simulink model "quad_control"  (R2014b)
settings: Solver=ode3  StartTime=0.0  StopTime=100  FixedStep=0.01  RelTol=1e-3
values from neighbouring files (symbols this model uses):
  g = 9.8    [init.m]
  m = 0.18    [init.m]
undefined symbols (not defined in the file or in its folder): attitude_control, commanded_cord, model, position_control
libraries: simulink x2
settings Model: CovSFcnEnable=on  Creator=smishra  LastModifiedBy=smishra
settings DebuggingCC: SolverPrmCheckMsg=none  FrameProcessingCompatibilityMsg=error

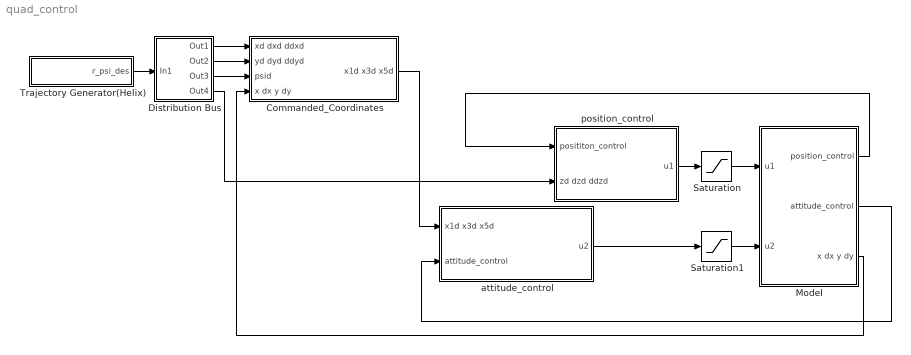
== system quad_control ==
  Commanded_Coordinates : Subsystem
  Distribution Bus : Subsystem
  Model : Subsystem
  Saturation : Saturate  UpperLimit=2*m*g  LowerLimit=0
  Saturation1 : Saturate  UpperLimit=0.2  LowerLimit=-0.2
  Trajectory Generator(Helix) : Subsystem
  attitude_control : Subsystem
  position_control : Subsystem
  wires:
  Model/1(position_control) -> position_control/1(posititon_control)
  Commanded_Coordinates/1(x1d x3d x5d) -> attitude_control/1(x1d x3d x5d)
  Model/2(attitude_control) -> attitude_control/2(attitude_control)
  Model/3(x dx y dy) -> Commanded_Coordinates/4(x dx y dy)
  position_control/1(u1) -> Saturation/1
  Saturation/1 -> Model/1(u1)
  Saturation1/1 -> Model/2(u2)
  attitude_control/1(u2) -> Saturation1/1
  Trajectory Generator(Helix)/1(r_psi_des) -> Distribution Bus/1(In1)
  Distribution Bus/1(Out1) -> Commanded_Coordinates/1(xd dxd ddxd)
  Distribution Bus/2(Out2) -> Commanded_Coordinates/2(yd dyd ddyd)
  Distribution Bus/3(Out3) -> Commanded_Coordinates/3(psid)
  Distribution Bus/4(Out4) -> position_control/2(zd dzd ddzd)

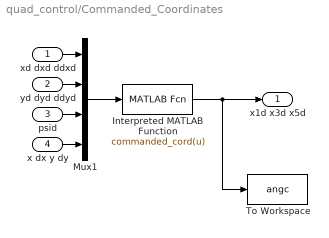
== system quad_control/Commanded_Coordinates ==
  xd dxd ddxd : Inport
  yd dyd ddyd : Inport  Port=2
  psid : Inport  Port=3
  x dx y dy : Inport  Port=4
  Interpreted MATLAB Function : MATLABFcn  MATLABFcn=commanded_cord(u)  OutputDimensions=3
  Mux1 : Mux
  To Workspace : ToWorkspace  VariableName=angc  SampleTime=-1
  x1d x3d x5d : Outport
  wires:
  yd dyd ddyd/1 -> Mux1/2
  xd dxd ddxd/1 -> Mux1/1
  psid/1 -> Mux1/3
  Interpreted MATLAB Function/1 -> To Workspace/1, x1d x3d x5d/1
  Mux1/1 -> Interpreted MATLAB Function/1
  x dx y dy/1 -> Mux1/4

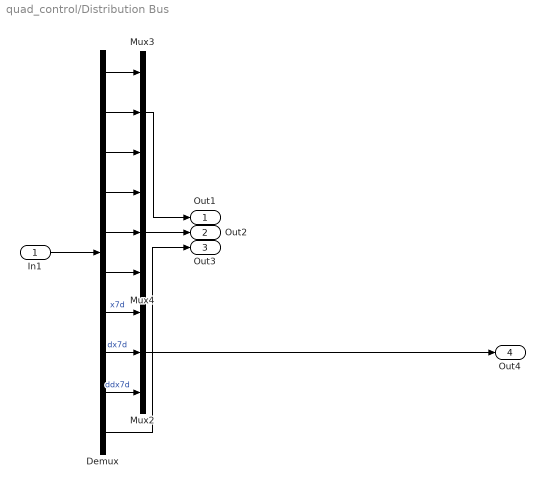
== system quad_control/Distribution Bus ==
  In1 : Inport
  Demux : Demux  Outputs=10
  Mux2 : Mux  Inputs=3
  Mux3 : Mux  Inputs=3
  Mux4 : Mux  Inputs=3
  Out1 : Outport
  Out2 : Outport  Port=2
  Out3 : Outport  Port=3
  Out4 : Outport  Port=4
  wires:
  Demux/10 -> Out3/1
  Mux4/1 -> Out2/1
  Mux3/1 -> Out1/1
  In1/1 -> Demux/1
  Demux/5 -> Mux4/2
  Demux/6 -> Mux4/3
  Demux/4 -> Mux4/1
  Demux/3 -> Mux3/3
  Demux/2 -> Mux3/2
  Demux/1 -> Mux3/1
  Mux2/1 -> Out4/1
  Demux/9 -> Mux2/3  "ddx7d"
  Demux/8 -> Mux2/2  "dx7d"
  Demux/7 -> Mux2/1  "x7d"

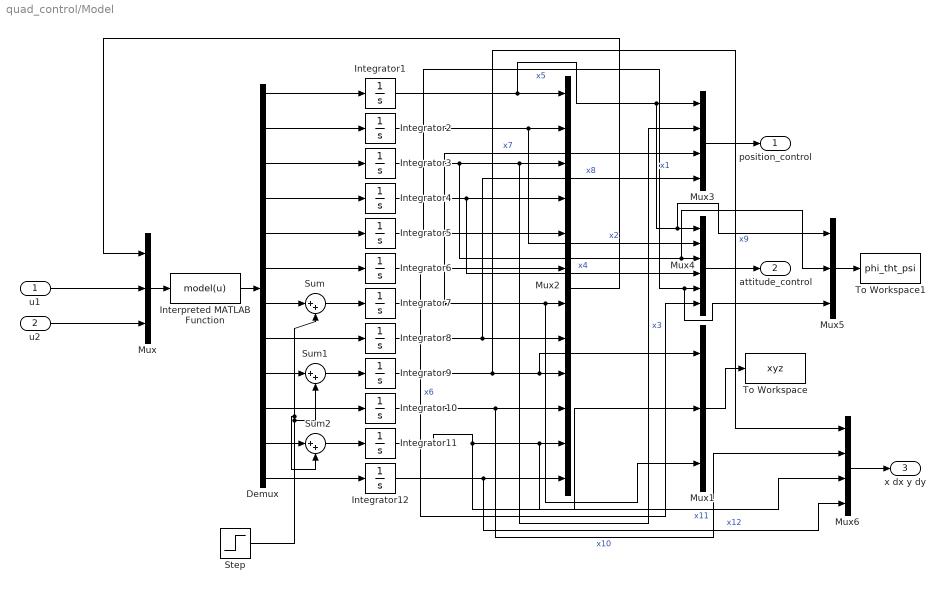
== system quad_control/Model ==
  u1 : Inport
  u2 : Inport  Port=2
  Demux : Demux  Outputs=12
  Integrator{1..6,8..10,12} (10 alike) : Integrator
  Integrator11 : Integrator  InitialCondition=8
  Integrator7 : Integrator  InitialCondition=-8
  Interpreted MATLAB Function : MATLABFcn  MATLABFcn=model(u)  OutputDimensions=12
  Mux : Mux  Inputs=3
  Mux1 : Mux  Inputs=3
  Mux2 : Mux  Inputs=12
  Mux3 : Mux
  Mux4 : Mux  Inputs=6
  Mux5 : Mux  Inputs=3
  Mux6 : Mux
  Step : Step  Time=25  After=5  SampleTime=0
  Sum : Sum  Inputs=|++
  Sum1 : Sum  Inputs=|++
  Sum2 : Sum  Inputs=|++
  To Workspace : ToWorkspace  VariableName=xyz  SampleTime=-1
  To Workspace1 : ToWorkspace  VariableName=phi_tht_psi  SampleTime=-1
  position_control : Outport
  attitude_control : Outport  Port=2
  x dx y dy : Outport  Port=3
  wires:
  Interpreted MATLAB Function/1 -> Demux/1
  Demux/1 -> Integrator1/1
  Demux/2 -> Integrator2/1
  Demux/3 -> Integrator3/1
  Demux/4 -> Integrator4/1
  Demux/5 -> Integrator5/1
  Demux/6 -> Integrator6/1
  Demux/8 -> Integrator8/1
  Demux/10 -> Integrator10/1
  Demux/12 -> Integrator12/1
  Integrator1/1 -> Mux5/1, Mux4/1, Mux3/1, Mux2/1  "x1"
  Integrator2/1 -> Mux4/2, Mux2/2  "x2"
  Integrator3/1 -> Mux5/2, Mux4/3, Mux3/2, Mux2/3  "x3"
  Integrator4/1 -> Mux4/4, Mux2/4  "x4"
  Integrator5/1 -> Mux5/3, Mux4/5, Mux2/5  "x5"
  Integrator6/1 -> Mux4/6, Mux2/6  "x6"
  Integrator7/1 -> Mux2/7, Mux1/3, Mux3/3  "x7"
  Integrator8/1 -> Mux3/4, Mux2/8  "x8"
  Integrator9/1 -> Mux6/1, Mux1/1, Mux2/9  "x9"
  Integrator10/1 -> Mux6/2, Mux2/10  "x10"
  Integrator11/1 -> Mux6/3, Mux1/2, Mux2/11  "x11"
  Integrator12/1 -> Mux6/4, Mux2/12  "x12"
  Mux/1 -> Interpreted MATLAB Function/1
  Mux2/1 -> Mux/1
  u1/1 -> Mux/2
  u2/1 -> Mux/3
  Mux1/1 -> To Workspace/1
  Mux3/1 -> position_control/1
  Mux4/1 -> attitude_control/1
  Mux5/1 -> To Workspace1/1
  Mux6/1 -> x dx y dy/1
  Demux/7 -> Sum/1
  Sum/1 -> Integrator7/1
  Demux/9 -> Sum1/1
  Sum1/1 -> Integrator9/1
  Demux/11 -> Sum2/1
  Sum2/1 -> Integrator11/1
  Step/1 -> Sum/2, Sum2/2, Sum1/2

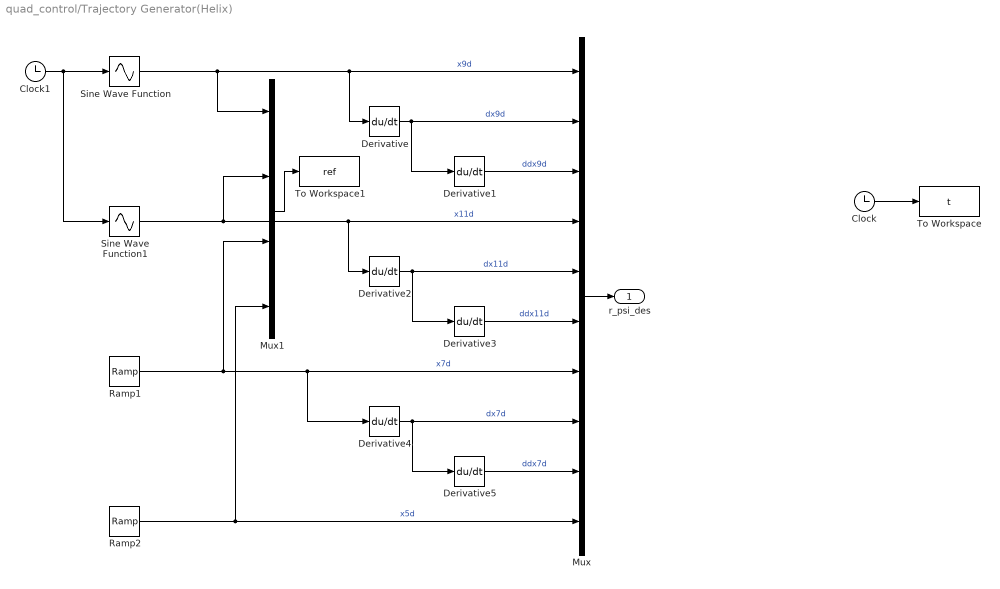
== system quad_control/Trajectory Generator(Helix) ==
  Clock : Clock
  Clock1 : Clock
  Derivative{,1..5} (6 alike) : Derivative
  Mux : Mux  Inputs=10
  Mux1 : Mux
  Ramp1 : simulink/Sources/Ramp  slope=0.2  start=0  X0=-8
  Ramp2 : simulink/Sources/Ramp  slope=0  start=0  X0=0
  Sine Wave Function : Sin  TimeSource=Use external signal  Amplitude=8  Frequency=0.1  SampleTime=0
  Sine Wave Function1 : Sin  TimeSource=Use external signal  Amplitude=8  Frequency=0.1  Phase=pi/2  SampleTime=0
  To Workspace : ToWorkspace  VariableName=t  SampleTime=-1
  To Workspace1 : ToWorkspace  VariableName=ref  SampleTime=-1
  r_psi_des : Outport
  wires:
  Derivative2/1 -> Mux/5, Derivative3/1  "dx11d"
  Derivative4/1 -> Mux/8, Derivative5/1  "dx7d"
  Derivative/1 -> Mux/2, Derivative1/1  "dx9d"
  Derivative1/1 -> Mux/3  "ddx9d"
  Derivative3/1 -> Mux/6  "ddx11d"
  Derivative5/1 -> Mux/9  "ddx7d"
  Sine Wave Function/1 -> Mux1/1, Mux/1, Derivative/1  "x9d"
  Ramp2/1 -> Mux1/4, Mux/10  "x5d"
  Mux/1 -> r_psi_des/1
  Clock/1 -> To Workspace/1
  Clock1/1 -> Sine Wave Function1/1, Sine Wave Function/1
  Ramp1/1 -> Mux1/3, Derivative4/1, Mux/7  "x7d"
  Mux1/1 -> To Workspace1/1
  Sine Wave Function1/1 -> Mux1/2, Derivative2/1, Mux/4  "x11d"

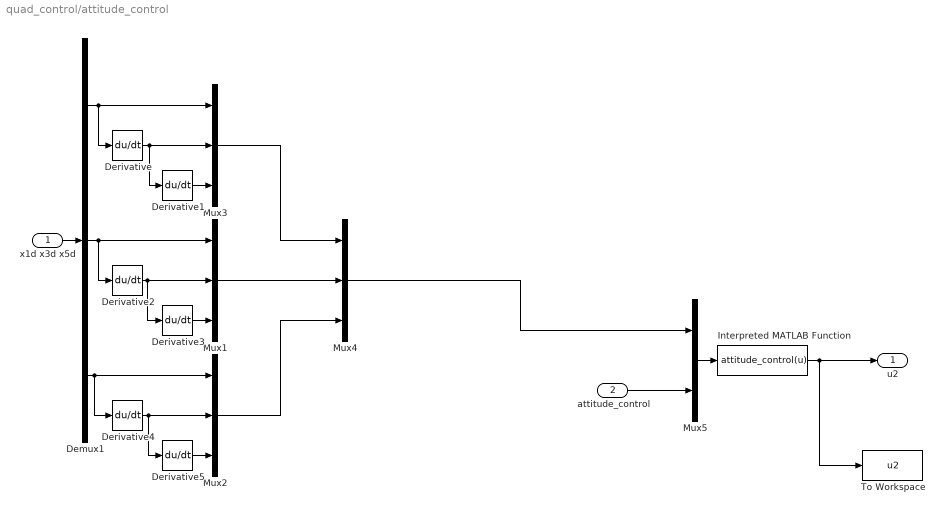
== system quad_control/attitude_control ==
  x1d x3d x5d : Inport
  attitude_control : Inport  Port=2
  Demux1 : Demux  Outputs=3
  Derivative{,1..5} (6 alike) : Derivative
  Interpreted MATLAB Function : MATLABFcn  MATLABFcn=attitude_control(u)  OutputDimensions=3
  Mux{1..4} (4 alike) : Mux  Inputs=3
  Mux5 : Mux  Inputs=2
  To Workspace : ToWorkspace  VariableName=u2  SampleTime=-1
  u2 : Outport
  wires:
  Demux1/1 -> Derivative/1, Mux3/1
  x1d x3d x5d/1 -> Demux1/1
  Mux5/1 -> Interpreted MATLAB Function/1
  Interpreted MATLAB Function/1 -> To Workspace/1, u2/1
  Derivative/1 -> Derivative1/1, Mux3/2
  Derivative1/1 -> Mux3/3
  Demux1/2 -> Derivative2/1, Mux1/1
  Derivative2/1 -> Mux1/2, Derivative3/1
  Derivative3/1 -> Mux1/3
  Derivative4/1 -> Mux2/2, Derivative5/1
  Derivative5/1 -> Mux2/3
  Demux1/3 -> Derivative4/1, Mux2/1
  Mux3/1 -> Mux4/1
  Mux1/1 -> Mux4/2
  Mux2/1 -> Mux4/3
  Mux4/1 -> Mux5/1
  attitude_control/1 -> Mux5/2

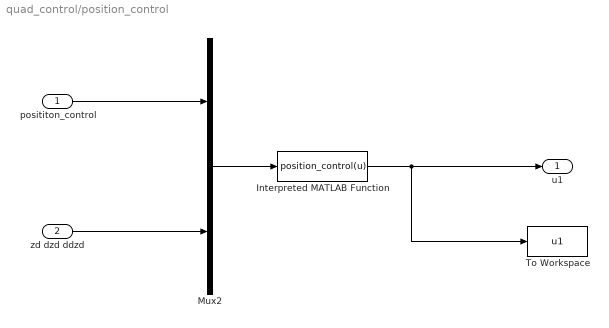
== system quad_control/position_control ==
  posititon_control : Inport
  zd dzd ddzd : Inport  Port=2
  Interpreted MATLAB Function : MATLABFcn  MATLABFcn=position_control(u)  OutputDimensions=1
  Mux2 : Mux  Inputs=2
  To Workspace : ToWorkspace  VariableName=u1  SampleTime=-1
  u1 : Outport
  wires:
  Interpreted MATLAB Function/1 -> To Workspace/1, u1/1
  Mux2/1 -> Interpreted MATLAB Function/1
  posititon_control/1 -> Mux2/1
  zd dzd ddzd/1 -> Mux2/2
